simulink model "lookupTableDynamic_TestGen8"  (R2017b)
settings: Solver=FixedStepDiscrete  StartTime=0.0  StopTime=10.0  RelTol=1e-3
undefined symbols (not defined in the file): Block_TestLib, reset
libraries: simulink x1
settings Model: Creator=ktrinh  LastModifiedBy=ktrinh
settings DebuggingCC: ParameterOverflowMsg=none

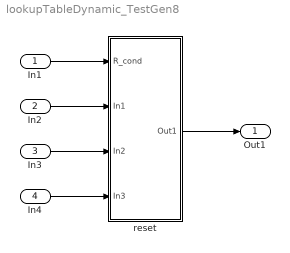
== system lookupTableDynamic_TestGen8 ==
  In1 : Inport
  In2 : Inport  Port=2
  In3 : Inport  Port=3
  In4 : Inport  Port=4
  reset : Subsystem  AncestorBlock=Block_TestLib/reset
  Out1 : Outport
  wires:
  In1/1 -> reset/1(R_cond)
  In2/1 -> reset/2(In1)
  In3/1 -> reset/3(In2)
  In4/1 -> reset/4(In3)
  reset/1(Out1) -> Out1/1

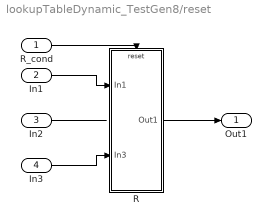
== system lookupTableDynamic_TestGen8/reset ==
  R_cond : Inport  OutDataTypeStr=boolean
  In1 : Inport  Port=2
  In2 : Inport  Port=3
  In3 : Inport  Port=4
  R : Subsystem  TreatAsAtomicUnit=on
  Out1 : Outport
  wires:
  R_cond/1 -> R/Reset
  In1/1 -> R/1(In1)
  In2/1 -> ?
  In3/1 -> R/2(In3)
  R/1(Out1) -> Out1/1

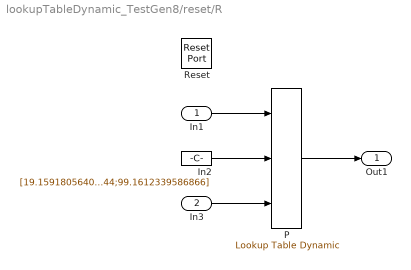
== system lookupTableDynamic_TestGen8/reset/R ==
  In1 : Inport  OutMin=17.1592  OutMax=101  OutDataTypeStr=uint32  PortDimensions=1
  In3 : Inport  Port=2  PortDimensions=5
  Reset : ResetPort  DisableCoverage=on
  In2 : Constant  Value=[19.1591805640469;37.9765202816717;44.9998784363792;56.7039267287644;99.1612339586866]  OutDataTypeStr=uint32
  P : simulink/Lookup Tables/Lookup Table Dynamic  LookUpMeth=Interpolation-Extrapolation  OutDataType=fixdt('uint32')  OutScaling=[]  OutputDataTypeScalingMode=Specify via dialog  OutDataTypeStr=uint32  RndMeth=Convergent  DoSatur=off
      settings: SourceProductName=Simulink
  Out1 : Outport
  wires:
  In1/1 -> P/1
  In2/1 -> P/2
  In3/1 -> P/3
  P/1 -> Out1/1
